simulink model "k1vistmsx"  (Simulink 8.6)
settings: Solver=ode45  StartTime=0.0  StopTime=10.0  RelTol=1e-3
libraries: cdsEpicsOut x52, cdsFilt x39, cdsTP x30, cdsFiltCtrl x26, cdsRms x12, cdsEpicsIn x10, cdsMuxMatrix x6, cdsCDI64 x2, cdsCDO64 x2, cdsIPCx x2, STATE_BIO_MASTER x2, cdsEpicsBinIn x2
(part 1 of 7)
settings Model: Creator=controls  LastModifiedBy=controls
settings OptimizationCC: InitFltsAndDblsToZero=on
settings DebuggingCC: FcnCallInpInsideContextMsg=EnableAllAsWarning  AllowSymbolicDim=on  StrictBusMsg=Warning

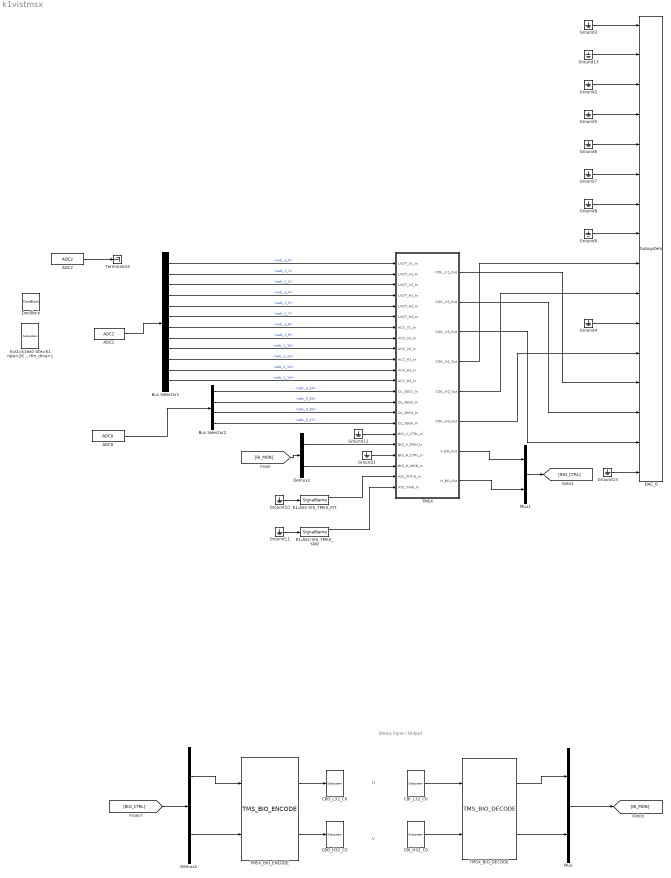
== system k1vistmsx ==
  note: Binary Input / Output
  note: H
  note: V
  ADC0 : cdsAdcx0/ADC0  Tag=cdsAdc  Description=|
      | type-GSC_16AI64SSA
      | card_num=0
      settings: AttributesFormatString=%<Description>\n%<Tag>
  ADC1 : cdsAdcx1/ADC1  Tag=cdsAdc  Description=|
      | type-GSC_16AI64SSA
      | card_num=1
      settings: AttributesFormatString=%<Description>\n%<Tag>
  ADC2 : cdsAdcx2/ADC2  Tag=cdsAdc  Description=|
      | type-GSC_16AI64SSA
      | card_num=2
      settings: AttributesFormatString=%<Description>\n%<Tag>
  Bus Selector1 : BusSelector  Description=ADC Selector  OutputSignals=adc_1_0,adc_1_1,adc_1_2,adc_1_4,adc_1_5,adc_1_7,adc_1_8,adc_1_9,adc_1_10,adc_1_12,adc_1_13,adc_1_14
      settings: AttributesFormatString=%<Description>
  Bus Selector2 : BusSelector  Description=ADC Selector  OutputSignals=adc_0_24,adc_0_25,adc_0_26,adc_0_27
      settings: AttributesFormatString=%<Description>
  CBI_H32_C0 : cdsCDI64/Subsystem  Tag=cdsCDI64  Description=card_num=1
      settings: AttributesFormatString=%<Tag>\n%<Description>
  CBI_L32_C0 : cdsCDI64/Subsystem  Tag=cdsCDI64  Description=card_num=0
      settings: AttributesFormatString=%<Tag>\n%<Description>
  CBO_H32_C0 : cdsCDO64/Subsystem  Tag=cdsCDO64  Description=card_num=1
      settings: AttributesFormatString=%<Tag>\n%<Description>
  CBO_L32_C0 : cdsCDO64/Subsystem  Tag=cdsCDO64  Description=card_num=0
      settings: AttributesFormatString=%<Tag>\n%<Description>
  DAC_0 : dac/Subsystem  Description=|
      | type=GSC_16AO16,
      | card_num=0
      settings: AttributesFormatString=%<Description>
  Demux1 : Demux  Outputs=2
  Demux2 : Demux  Outputs=2
  DocBlock : simulink/Model-Wide Utilities/DocBlock  DocumentType=Text
  Ground{1..13,15} (14 alike) : Ground
  K1:ASC-VIS_TMSX_PIT : cdsIPCx/SignalName  Tag=cdsIPCx_RFM  Description=card=0
      settings: AttributesFormatString=%<Description>\n%<Tag>
  K1:ASC-VIS_TMSX_YAW : cdsIPCx/SignalName  Tag=cdsIPCx_RFM  Description=card=0
      settings: AttributesFormatString=%<Description>\n%<Tag>
  Mux : Mux  Inputs=2
  Mux1 : Mux  Inputs=2
  TMSX : Subsystem  AncestorBlock=VIS_TMS_LIB/TMS_VIS
  TMSX_BIO_DECODE : VIS_TMS_LIB/TMS_BIO_DECODE
  TMSX_BIO_ENCODE : VIS_TMS_LIB/TMS_BIO_ENCODE
  Terminator4 : Terminator
  host=k1ex0 site=K1 rate=2K dcuid=107 specific_cpu=7 adcSlave=1 no_rfm_dma=1 : cdsParameters/Subsystem  Tag=cdsParameters  Description=|
      | Purpose:                                                                                                                                                                                                                                
      |                                                                                                                                                                                                                                         
      | Provide system parameters to the FE code generator to properly configure the generated EPICS names, rep rate of the FE controller, and the Data Acquisition node ID for proper storage of data from this FE controller.                 
      |                                                                                                                                                                                                                                         
      | Useage:                                                                                                                                                                                                                                 
      |                                                                                                                                                                                                                                         
      | The part NAME field is used to identify the FE parameters. It must be of the form:                                                                                                                                                      
      |                                                                                                                                                                                                                                         
      | site=                                                                                                                                                                                                                                   
      | rate=                                                                                                                                                                                                                                   
      | dcuid=                                                                                                                                                                                                                                  
      |                                                                                                                                                                                                                                         
      | Where:                                                                                                                                                                                                                                  
      |                                                                                                                                                                                                                                         
      | site= argument may be H1, H2, L1, M1, G1, either as a single argument or multiple, for example site=H1,H2. These are the only names allowed. These will become the first two characters of all EPICS and signal names (for example G1:).
      |                                                                                                                                                                                                                                         
      | rate= may be 2K, 16K, 32K, or 64K                                                                                                                                                                                                       
      |                                                                                                                                                                                                                                         
      | dcuid= is site specific ie it must be unique at each site.
      settings: AttributesFormatString=%<Tag>
  wires:
  ADC0/1 -> Bus Selector2/1
  Bus Selector1/10 -> TMSX/10(ACC_H1_In)  "<adc_1_12>"
  Bus Selector1/11 -> TMSX/11(ACC_H2_In)  "<adc_1_13>"
  Bus Selector1/12 -> TMSX/12(ACC_H3_In)  "<adc_1_14>"
  TMSX_BIO_ENCODE/1 -> CBO_L32_C0/1
  CBI_L32_C0/1 -> TMSX_BIO_DECODE/1
  TMSX_BIO_DECODE/2 -> Mux/2
  TMSX_BIO_DECODE/1 -> Mux/1
  Mux/1 -> [BI_MON]
  [BIO_CTRL] -> Demux1/1
  TMSX_BIO_ENCODE/2 -> CBO_H32_C0/1
  Demux1/1 -> TMSX_BIO_ENCODE/1
  Demux1/2 -> TMSX_BIO_ENCODE/2
  CBI_H32_C0/1 -> TMSX_BIO_DECODE/2
  [BI_MON] -> Demux2/1
  TMSX/7(V_BO_Out) -> Mux1/1
  TMSX/8(H_BO_Out) -> Mux1/2
  Mux1/1 -> [BIO_CTRL]
  TMSX/1(COIL_V1_Out) -> DAC_0/13
  TMSX/2(COIL_V2_Out) -> DAC_0/14
  TMSX/3(COIL_V3_Out) -> DAC_0/15
  Demux2/1 -> TMSX/18(BIO_V_MON_In)
  Ground1/1 -> TMSX/19(BIO_H_CTRL_In)
  Ground12/1 -> TMSX/17(BIO_V_CTRL_In)
  Demux2/2 -> TMSX/20(BIO_H_MON_In)
  Bus Selector1/1 -> TMSX/1(LVDT_V1_In)  "<adc_1_0>"
  Bus Selector1/2 -> TMSX/2(LVDT_V2_In)  "<adc_1_1>"
  Bus Selector1/3 -> TMSX/3(LVDT_V3_In)  "<adc_1_2>"
  Bus Selector1/4 -> TMSX/4(LVDT_H1_In)  "<adc_1_4>"
  Bus Selector1/5 -> TMSX/5(LVDT_H2_In)  "<adc_1_5>"
  Bus Selector1/6 -> TMSX/6(LVDT_H3_In)  "<adc_1_7>"
  Bus Selector1/7 -> TMSX/7(ACC_V1_In)  "<adc_1_8>"
  Bus Selector1/8 -> TMSX/8(ACC_V2_In)  "<adc_1_9>"
  Bus Selector1/9 -> TMSX/9(ACC_V3_In)  "<adc_1_10>"
  Ground3/1 -> DAC_0/1
  Ground2/1 -> DAC_0/3
  Bus Selector2/1 -> TMSX/13(OL_SEG1_In)  "<adc_0_24>"
  Bus Selector2/2 -> TMSX/14(OL_SEG2_In)  "<adc_0_25>"
  Bus Selector2/3 -> TMSX/15(OL_SEG3_In)  "<adc_0_26>"
  Bus Selector2/4 -> TMSX/16(OL_SEG4_In)  "<adc_0_27>"
  Ground13/1 -> DAC_0/2
  Ground7/1 -> DAC_0/6
  Ground6/1 -> DAC_0/5
  Ground5/1 -> DAC_0/4
  Ground8/1 -> DAC_0/7
  Ground9/1 -> DAC_0/8
  TMSX/4(COIL_H1_Out) -> DAC_0/9
  TMSX/5(COIL_H2_Out) -> DAC_0/10
  Ground4/1 -> DAC_0/11
  TMSX/6(COIL_H3_Out) -> DAC_0/12
  Ground15/1 -> DAC_0/16
  ADC2/1 -> Terminator4/1
  ADC1/1 -> Bus Selector1/1
  Ground10/1 -> K1:ASC-VIS_TMSX_PIT/1
  Ground11/1 -> K1:ASC-VIS_TMSX_YAW/1
  K1:ASC-VIS_TMSX_PIT/1 -> TMSX/21(ASC_PITCH_In)
  K1:ASC-VIS_TMSX_YAW/1 -> TMSX/22(ASC_YAW_In)

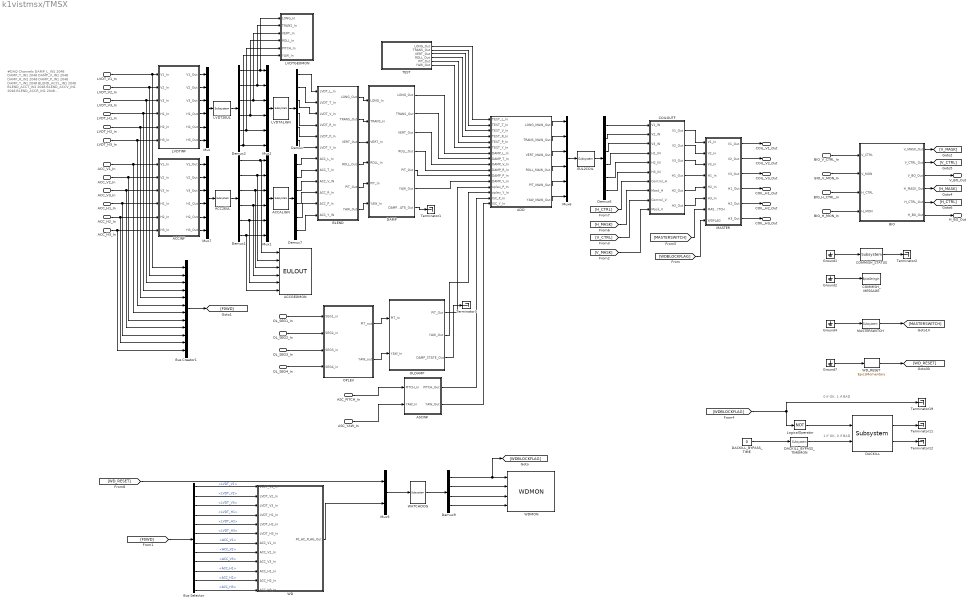
== system k1vistmsx/TMSX ==
  note: #DAQ Channels
      | DAMP_L_IN1 2048
      | DAMP_T_IN1 2048
      | DAMP_V_IN1 2048
      | DAMP_R_IN1 2048
      | DAMP_P_IN1 2048
      | DAMP_Y_IN1 2048
      | BLEND_ACCL_IN1 2048
      | BLEND_ACCT_IN1 2048
      | BLEND_ACCV_IN1 2048
      | BLEND_ACCR_IN1 2048
      | BLEND_ACCP_IN1 2048
      | BLEND_ACCY_IN1 2048
      | BLEND_LVDTL_IN1 2048
      | BLEND_LVDTT_IN1 2048
      | BLEND_LVDTV_IN1 2048
      | BLEND_LVDTR_IN1 2048
      | BLEND_LVDTP_IN1 2048
      | BLEND_LVDTY_IN1 2048
  note: 1 if OK, 0 if BAD
  note: 0 if OK, 1 if BAD
  LVDT_V1_In : Inport
  LVDT_V2_In : Inport  Port=2
  LVDT_V3_In : Inport  Port=3
  LVDT_H1_In : Inport  Port=4
  LVDT_H2_In : Inport  Port=5
  LVDT_H3_In : Inport  Port=6
  ACC_V1_In : Inport  Port=7
  ACC_V2_In : Inport  Port=8
  ACC_V3_In : Inport  Port=9
  ACC_H1_In : Inport  Port=10
  ACC_H2_In : Inport  Port=11
  ACC_H3_In : Inport  Port=12
  OL_SEG1_In : Inport  Port=13
  OL_SEG2_In : Inport  Port=14
  OL_SEG3_In : Inport  Port=15
  OL_SEG4_In : Inport  Port=16
  BIO_V_CTRL_In : Inport  Port=17
  BIO_V_MON_In : Inport  Port=18
  BIO_H_CTRL_In : Inport  Port=19
  BIO_H_MON_In : Inport  Port=20
  ASC_PITCH_In : Inport  Port=21
  ASC_YAW_In : Inport  Port=22
  ACC2EUL : cdsMuxMatrix/Subsystem  Tag=cdsMuxMatrix  Description=|
      | ADL=SUS_INMATRIX.adl 
      | SCRIPT=generate_KisselButton.py 4 5 #CHANNEL# > #TARGET_DIR#/#FULL_PART_NAME#_KB.adl
      settings: AttributesFormatString=%<Tag>
  ACCALIGN : cdsMuxMatrix/Subsystem  Tag=cdsMuxMatrix  Description=Any size matrix. Inputs and outputs must be connected using Mux and Demux parts.
      settings: AttributesFormatString=%<Tag>
  ACCGEOMON : VIS_LIB/EULOUT
  ACCINF : Subsystem
  ADD : Subsystem
  ASCINF : Subsystem
  BIO : Subsystem
  BLEND : Subsystem
  Bus Creator1 : BusCreator  Inputs='LVDT_H1','LVDT_H2','LVDT_H3','LVDT_V1','LVDT_V2','LVDT_V3','ACC_H1','ACC_H2','ACC_H3','ACC_V1','ACC_V2','ACC_V3'
  Bus Selector : BusSelector  OutputSignals=LVDT_V1,LVDT_V2,LVDT_V3,LVDT_H1,LVDT_H2,LVDT_H3,ACC_V1,ACC_V2,ACC_V3,ACC_H1,ACC_H2,ACC_H3
  COILOUTF : Subsystem
  COMMISH_MESSAGE : cdsEpicsStringIn/EpicsStringIn  Tag=cdsEpicsStringIn  Description=cdsEpicsStringIn
      settings: AttributesFormatString=%<Tag>
  COMMISH_STATUS : cdsEpicsBinIn/Subsystem  Tag=cdsEpicsBinIn  Description=|
      | Purpose:                                                                            
      | Create an EPICS binary (0 or 1) input channel to the FE realtime controls.          
      |                                                                                     
      | Operation:                                                                          
      | Outputs value from an EPICS ai record. Value is binary input (bi Epics record type).
      |                                                                                     
      | Usage:                                                                              
      | Name the part with the desired EPICS channel name.
      settings: AttributesFormatString=%<Tag>
  DACKILL : cdsDacKill/Subsystem  Description=cdsDacKill
      settings: AttributesFormatString=%<Description>
  DACKILL_BYPASS_TIME : Constant  Value=0
  DACKILL_BYPASS_TIMEMON : cdsEpicsOut/Subsystem  Tag=cdsEpicsOutput  Description=|
      | Purpose:                                          
      | Output a FE signal to an EPICS channel.           
      |                                                   
      | Operation:                                        
      | Takes input value and passes it to EPICS record.  
      |                                                   
      | Usage:                                            
      | Name the part with the desired EPICS rrecord name.
      settings: AttributesFormatString=%<Tag>
  DAMP : Subsystem
  Demux{,1..2,6..7} (5 alike) : Demux  Outputs=6
  Demux9 : Demux
  EUL2COIL : cdsMuxMatrix/Subsystem  Tag=cdsMuxMatrix  Description=|
      | ADL=SUS_INMATRIX.adl 
      | SCRIPT=generate_KisselButton.py 4 5 #CHANNEL# > #TARGET_DIR#/#FULL_PART_NAME#_KB.adl
      settings: AttributesFormatString=%<Tag>
  Ground{1..2,4,7} (4 alike) : Ground
  LVDT2EUL : cdsMuxMatrix/Subsystem  Tag=cdsMuxMatrix  Description=|
      | ADL=SUS_INMATRIX.adl 
      | SCRIPT=generate_KisselButton.py 4 5 #CHANNEL# > #TARGET_DIR#/#FULL_PART_NAME#_KB.adl
      settings: AttributesFormatString=%<Tag>
  LVDTALIGN : cdsMuxMatrix/Subsystem  Tag=cdsMuxMatrix  Description=Any size matrix. Inputs and outputs must be connected using Mux and Demux parts.
      settings: AttributesFormatString=%<Tag>
  LVDTGEOMON : Subsystem  AncestorBlock=VIS_LIB/EULOUT
  LVDTINF : Subsystem
  LogicalOperator : Logic  Operator=NOT  AllPortsSameDT=off  OutDataTypeStr=boolean
  MASTER : Subsystem
  MASTERSWITCH : cdsEpicsBinIn/Subsystem  Tag=cdsEpicsBinIn  Description=|
      | Purpose:                                                                            
      | Create an EPICS binary (0 or 1) input channel to the FE realtime controls.          
      |                                                                                     
      | Operation:                                                                          
      | Outputs value from an EPICS ai record. Value is binary input (bi Epics record type).
      |                                                                                     
      | Usage:                                                                              
      | Name the part with the desired EPICS channel name.
      settings: AttributesFormatString=%<Tag>
  Mux{,1..2,6..7} (5 alike) : Mux  Inputs=6
  Mux9 : Mux  Inputs=2
  OLDAMP : Subsystem
  OPLEV : Subsystem
  TEST : Subsystem
  Terminator{1..3,11..12,19} (6 alike) : Terminator
  WATCHDOG : cdsFunctionCall/Subsystem  Tag=cdsFunctionCall  Description=inline OSEMWATCHDOG /opt/rtcds/userapps/release/vis/common/src/WATCHDOG.c
      settings: AttributesFormatString=%<Tag>\n%<Description>
  WD : Subsystem
  WDMON : SIXOSEM_F_STAGE_MASTER/SIXOSEM_F_STAGE_MASTER/WDMON
  WD_RESET : cdsEpicsMomentary/EpicsMomentary  Tag=cdsEpicsMomentary
      settings: AttributesFormatString=%<Tag>
  COIL_V1_Out : Outport
  COIL_V2_Out : Outport  Port=2
  COIL_V3_Out : Outport  Port=3
  COIL_H1_Out : Outport  Port=4
  COIL_H2_Out : Outport  Port=5
  COIL_H3_Out : Outport  Port=6
  V_BO_Out : Outport  Port=7
  H_BO_Out : Outport  Port=8
  wires:
  ASCINF/2(YAW_Out) -> ADD/16(ISC_Y_In)
  ASCINF/1(PITCH_Out) -> ADD/15(ISC_P_In)
  ASC_YAW_In/1 -> ASCINF/2(YAW_In)
  ASC_PITCH_In/1 -> ASCINF/1(PITCH_In)
  DAMP/3(VERT_Out) -> ADD/9(DAMP_V_In)
  DAMP/2(TRANS_Out) -> ADD/8(DAMP_T_In)
  DAMP/1(LONG_Out) -> ADD/7(DAMP_L_In)
  TEST/3(VERT_Out) -> ADD/3(TEST_V_In)
  TEST/2(TRANS_Out) -> ADD/2(TEST_T_In)
  TEST/1(LONG_Out) -> ADD/1(TEST_L_In)
  DAMP/7(DAMP_STATE_Out) -> Terminator1/1
  [WDBLOCKFLAG] -> MASTER/8(WDFLAG)
  Bus Creator1/1 -> [F0WD]
  WATCHDOG/1 -> Demux9/1
  Mux9/1 -> WATCHDOG/1
  Demux9/4 -> WDMON/4
  Demux9/3 -> WDMON/3
  Demux9/2 -> WDMON/2
  Demux9/1 -> WDMON/1, [WDBLOCKFLAG]
  [F0WD] -> Bus Selector/1
  WD/1(F0_AC_FLAG_Out) -> Mux9/2
  [WD_RESET] -> Mux9/1
  [MASTERSWITCH] -> MASTER/7(MASTERSWITCH)
  EUL2COIL/1 -> Demux6/1
  Mux6/1 -> EUL2COIL/1
  Demux/3 -> BLEND/3(LVDT_V_In)
  Demux/2 -> BLEND/2(LVDT_T_In)
  Demux/1 -> BLEND/1(LVDT_L_In)
  ACC2EUL/1 -> Demux1/1
  Mux7/1 -> ACC2EUL/1
  LVDT2EUL/1 -> Demux2/1
  Mux/1 -> LVDT2EUL/1
  Demux/4 -> BLEND/4(LVDT_R_In)
  Demux/5 -> BLEND/5(LVDT_P_In)
  Demux/6 -> BLEND/6(LVDT_Y_In)
  Demux7/6 -> BLEND/12(ACC_Y_IN)
  Demux7/5 -> BLEND/11(ACC_P_In)
  Demux7/4 -> BLEND/10(ACC_R_In)
  Demux7/3 -> BLEND/9(ACC_V_IN)
  Demux7/2 -> BLEND/8(ACC_T_In)
  Demux7/1 -> BLEND/7(ACC_L_In)
  BLEND/1(LONG_Out) -> DAMP/1(LONG_In)
  BLEND/2(TRANS_Out) -> DAMP/2(TRANS_In)
  BLEND/3(VERT_Out) -> DAMP/3(VERT_In)
  BLEND/4(ROLL_Out) -> DAMP/4(ROLL_In)
  BLEND/5(PIT_Out) -> DAMP/5(PIT_In)
  BLEND/6(YAW_Out) -> DAMP/6(YAW_In)
  DAMP/4(ROLL_Out) -> ADD/10(DAMP_R_In)
  DAMP/5(PIT_Out) -> ADD/11(DAMP_P_In)
  DAMP/6(YAW_Out) -> ADD/12(DAMP_Y_In)
  TEST/4(ROLL_Out) -> ADD/4(TEST_R_In)
  TEST/5(PIT_Out) -> ADD/5(TEST_P_In)
  TEST/6(YAW_Out) -> ADD/6(TEST_Y_In)
  ADD/1(LONG_MAIN_Out) -> Mux6/1
  ADD/2(TRANS_MAIN_Out) -> Mux6/2
  ADD/3(VERT_MAIN_Out) -> Mux6/3
  ADD/4(ROLL_MAIN_Out) -> Mux6/4
  ADD/5(PIT_MAIN_Out) -> Mux6/5
  ADD/6(YAW_MAIN_Out) -> Mux6/6
  OL_SEG1_In/1 -> OPLEV/1(SEG1_in)
  OL_SEG2_In/1 -> OPLEV/2(SEG2_in)
  OL_SEG3_In/1 -> OPLEV/3(SEG3_in)
  OL_SEG4_In/1 -> OPLEV/4(SEG4_in)
  BIO/1(V_MASK_Out) -> [V_MASK]
  BIO/4(H_MASK_Out) -> [H_MASK]
  BIO/2(V_CTRL_Out) -> [V_CTRL]
  BIO/5(H_CTRL_Out) -> [H_CTRL]
  BIO/3(V_BO_Out) -> V_BO_Out/1
  BIO/6(H_BO_Out) -> H_BO_Out/1
  [H_CTRL] -> COILOUTF/7(Control_H)
  [H_MASK] -> COILOUTF/8(Mask_H)
  [V_CTRL] -> COILOUTF/9(Control_V)
  [V_MASK] -> COILOUTF/10(Mask_V)
  BIO_V_CTRL_In/1 -> BIO/1(V_CTRL)
  BIO_V_MON_In/1 -> BIO/2(V_MON)
  BIO_H_CTRL_In/1 -> BIO/3(H_CTRL)
  BIO_H_MON_In/1 -> BIO/4(H_MON)
  DACKILL/2 -> Terminator12/1
  DACKILL/1 -> Terminator11/1
  DACKILL_BYPASS_TIME/1 -> DACKILL_BYPASS_TIMEMON/1
  DACKILL_BYPASS_TIMEMON/1 -> DACKILL/2
  LogicalOperator/1 -> DACKILL/1
  [WDBLOCKFLAG] -> LogicalOperator/1, Terminator19/1
  Ground1/1 -> COMMISH_STATUS/1
  COMMISH_STATUS/1 -> Terminator2/1
  Ground2/1 -> COMMISH_MESSAGE/1
  MASTERSWITCH/1 -> [MASTERSWITCH]
  Ground4/1 -> MASTERSWITCH/1
  Ground7/1 -> WD_RESET/1
  WD_RESET/1 -> [WD_RESET]
  OPLEV/1(PIT_out) -> OLDAMP/1(PIT_In)
  OPLEV/2(YAW_out) -> OLDAMP/2(YAW_In)
  OLDAMP/1(PIT_Out) -> ADD/13(oplev_P_In)
  OLDAMP/2(YAW_Out) -> ADD/14(oplev_Y_In)
  OLDAMP/3(DAMP_STATE_Out) -> Terminator3/1
  LVDTINF/1(V1_Out) -> Mux/1
  LVDTINF/2(V2_Out) -> Mux/2
  LVDTINF/3(V3_Out) -> Mux/3
  LVDTINF/4(H1_Out) -> Mux/4
  LVDTINF/5(H2_Out) -> Mux/5
  LVDTINF/6(H3_Out) -> Mux/6
  ACCINF/1(V1_Out) -> Mux7/1
  ACCINF/2(V2_Out) -> Mux7/2
  ACCINF/3(V3_Out) -> Mux7/3
  ACCINF/4(H1_Out) -> Mux7/4
  ACCINF/5(H2_Out) -> Mux7/5
  ACCINF/6(H3_Out) -> Mux7/6
  LVDT_V1_In/1 -> LVDTINF/1(V1_In), Bus Creator1/1
  LVDT_V2_In/1 -> LVDTINF/2(V2_In), Bus Creator1/2
  LVDT_V3_In/1 -> LVDTINF/3(V3_In), Bus Creator1/3
  LVDT_H1_In/1 -> LVDTINF/4(H1_In), Bus Creator1/4
  LVDT_H2_In/1 -> LVDTINF/5(H2_In), Bus Creator1/5
  LVDT_H3_In/1 -> LVDTINF/6(H3_In), Bus Creator1/6
  ACC_V1_In/1 -> ACCINF/1(V1_In), Bus Creator1/7
  ACC_V2_In/1 -> ACCINF/2(V2_In), Bus Creator1/8
  ACC_V3_In/1 -> ACCINF/3(V3_In), Bus Creator1/9
  ACC_H1_In/1 -> ACCINF/4(H1_In), Bus Creator1/10
  ACC_H2_In/1 -> ACCINF/5(H2_In), Bus Creator1/11
  ACC_H3_In/1 -> ACCINF/6(H3_In), Bus Creator1/12
  Bus Selector/1 -> WD/1(LVDT_V1_In)  "<LVDT_V1>"
  Bus Selector/2 -> WD/2(LVDT_V2_In)  "<LVDT_V2>"
  Bus Selector/3 -> WD/3(LVDT_V3_In)  "<LVDT_V3>"
  Bus Selector/4 -> WD/4(LVDT_H1_In)  "<LVDT_H1>"
  Bus Selector/5 -> WD/5(LVDT_H2_In)  "<LVDT_H2>"
  Bus Selector/6 -> WD/6(LVDT_H3_In)  "<LVDT_H3>"
  Bus Selector/7 -> WD/7(ACC_V1_In)  "<ACC_V1>"
  Bus Selector/8 -> WD/8(ACC_V2_In)  "<ACC_V2>"
  Bus Selector/9 -> WD/9(ACC_V3_In)  "<ACC_V3>"
  Bus Selector/10 -> WD/10(ACC_H1_In)  "<ACC_H1>"
  Bus Selector/11 -> WD/11(ACC_H2_In)  "<ACC_H2>"
  Bus Selector/12 -> WD/12(ACC_H3_In)  "<ACC_H3>"
  Demux6/1 -> COILOUTF/1(V1_IN)
  Demux6/2 -> COILOUTF/2(V2_IN)
  Demux6/3 -> COILOUTF/3(V3_IN)
  Demux6/4 -> COILOUTF/4(H1_IN)
  Demux6/5 -> COILOUTF/5(H2_IN)
  Demux6/6 -> COILOUTF/6(H3_IN)
  COILOUTF/1(V1_Out) -> MASTER/1(V1_In)
  COILOUTF/2(V2_Out) -> MASTER/2(V2_In)
  COILOUTF/3(V3_Out) -> MASTER/3(V3_In)
  COILOUTF/4(H1_Out) -> MASTER/4(H1_In)
  COILOUTF/5(H2_Out) -> MASTER/5(H2_In)
  COILOUTF/6(H3_Out) -> MASTER/6(H3_In)
  MASTER/1(V1_Out) -> COIL_V1_Out/1
  MASTER/2(V2_Out) -> COIL_V2_Out/1
  MASTER/3(V3_Out) -> COIL_V3_Out/1
  MASTER/4(H1_Out) -> COIL_H1_Out/1
  MASTER/5(H2_Out) -> COIL_H2_Out/1
  MASTER/6(H3_Out) -> COIL_H3_Out/1
  Demux1/1 -> ACCGEOMON/1, Mux1/1
  ACCALIGN/1 -> Demux7/1
  Demux1/2 -> ACCGEOMON/2, Mux1/2
  Demux1/3 -> ACCGEOMON/3, Mux1/3
  Demux1/4 -> ACCGEOMON/4, Mux1/4
  Demux1/5 -> ACCGEOMON/5, Mux1/5
  Demux1/6 -> ACCGEOMON/6, Mux1/6
  Mux1/1 -> ACCALIGN/1
  Demux2/6 -> LVDTGEOMON/6(YAW_In), Mux2/6
  Demux2/4 -> LVDTGEOMON/4(ROLL_In), Mux2/4
  Demux2/3 -> LVDTGEOMON/3(VERT_In), Mux2/3
  Demux2/1 -> LVDTGEOMON/1(LONG_In), Mux2/1
  Mux2/1 -> LVDTALIGN/1
  LVDTALIGN/1 -> Demux/1
  Demux2/2 -> LVDTGEOMON/2(TRANS_In), Mux2/2
  Demux2/5 -> LVDTGEOMON/5(PITCH_In), Mux2/5

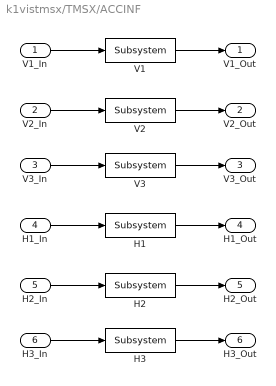
== system k1vistmsx/TMSX/ACCINF ==
  V1_In : Inport
  V2_In : Inport  Port=2
  V3_In : Inport  Port=3
  H1_In : Inport  Port=4
  H2_In : Inport  Port=5
  H3_In : Inport  Port=6
  H1 : cdsFilt/Subsystem  Tag=cdsFilt  Description=|
      | Purpose:                                                                                                                                                                                                                                  
      | Standard CDS IIR filter module.                                                                                                                                                                                                           
      |                                                                                                                                                                                                                                           
      | Operation:                                                                                                                                                                                                                                
      | Consists of 10 second order section IIR filters, plus a ramped gain stage. In FE code, also provides pre-defined test points and excitation channel inputs. The filter coefficients are defined in the LIGO system using the 'foton' tool.
      |                                                                                                                                                                                                                                           
      | Usage:                                                                                                                                                                                                                                    
      | Name the part with the desired filter module name.
      settings: AttributesFormatString=%<Tag>
  H2 : cdsFilt/Subsystem  Tag=cdsFilt  Description=|
      | Purpose:                                                                                                                                                                                                                                  
      | Standard CDS IIR filter module.                                                                                                                                                                                                           
      |                                                                                                                                                                                                                                           
      | Operation:                                                                                                                                                                                                                                
      | Consists of 10 second order section IIR filters, plus a ramped gain stage. In FE code, also provides pre-defined test points and excitation channel inputs. The filter coefficients are defined in the LIGO system using the 'foton' tool.
      |                                                                                                                                                                                                                                           
      | Usage:                                                                                                                                                                                                                                    
      | Name the part with the desired filter module name.
      settings: AttributesFormatString=%<Tag>
  H3 : cdsFilt/Subsystem  Tag=cdsFilt  Description=|
      | Purpose:                                                                                                                                                                                                                                  
      | Standard CDS IIR filter module.                                                                                                                                                                                                           
      |                                                                                                                                                                                                                                           
      | Operation:                                                                                                                                                                                                                                
      | Consists of 10 second order section IIR filters, plus a ramped gain stage. In FE code, also provides pre-defined test points and excitation channel inputs. The filter coefficients are defined in the LIGO system using the 'foton' tool.
      |                                                                                                                                                                                                                                           
      | Usage:                                                                                                                                                                                                                                    
      | Name the part with the desired filter module name.
      settings: AttributesFormatString=%<Tag>
  V1 : cdsFilt/Subsystem  Tag=cdsFilt  Description=|
      | Purpose:                                                                                                                                                                                                                                  
      | Standard CDS IIR filter module.                                                                                                                                                                                                           
      |                                                                                                                                                                                                                                           
      | Operation:                                                                                                                                                                                                                                
      | Consists of 10 second order section IIR filters, plus a ramped gain stage. In FE code, also provides pre-defined test points and excitation channel inputs. The filter coefficients are defined in the LIGO system using the 'foton' tool.
      |                                                                                                                                                                                                                                           
      | Usage:                                                                                                                                                                                                                                    
      | Name the part with the desired filter module name.
      settings: AttributesFormatString=%<Tag>
  V2 : cdsFilt/Subsystem  Tag=cdsFilt  Description=|
      | Purpose:                                                                                                                                                                                                                                  
      | Standard CDS IIR filter module.                                                                                                                                                                                                           
      |                                                                                                                                                                                                                                           
      | Operation:                                                                                                                                                                                                                                
      | Consists of 10 second order section IIR filters, plus a ramped gain stage. In FE code, also provides pre-defined test points and excitation channel inputs. The filter coefficients are defined in the LIGO system using the 'foton' tool.
      |                                                                                                                                                                                                                                           
      | Usage:                                                                                                                                                                                                                                    
      | Name the part with the desired filter module name.
      settings: AttributesFormatString=%<Tag>
  V3 : cdsFilt/Subsystem  Tag=cdsFilt  Description=|
      | Purpose:                                                                                                                                                                                                                                  
      | Standard CDS IIR filter module.                                                                                                                                                                                                           
      |                                                                                                                                                                                                                                           
      | Operation:                                                                                                                                                                                                                                
      | Consists of 10 second order section IIR filters, plus a ramped gain stage. In FE code, also provides pre-defined test points and excitation channel inputs. The filter coefficients are defined in the LIGO system using the 'foton' tool.
      |                                                                                                                                                                                                                                           
      | Usage:                                                                                                                                                                                                                                    
      | Name the part with the desired filter module name.
      settings: AttributesFormatString=%<Tag>
  V1_Out : Outport
  V2_Out : Outport  Port=2
  V3_Out : Outport  Port=3
  H1_Out : Outport  Port=4
  H2_Out : Outport  Port=5
  H3_Out : Outport  Port=6
  wires:
  H3/1 -> H3_Out/1
  H3_In/1 -> H3/1
  H2/1 -> H2_Out/1
  H2_In/1 -> H2/1
  H1/1 -> H1_Out/1
  H1_In/1 -> H1/1
  V3/1 -> V3_Out/1
  V3_In/1 -> V3/1
  V2/1 -> V2_Out/1
  V2_In/1 -> V2/1
  V1/1 -> V1_Out/1
  V1_In/1 -> V1/1

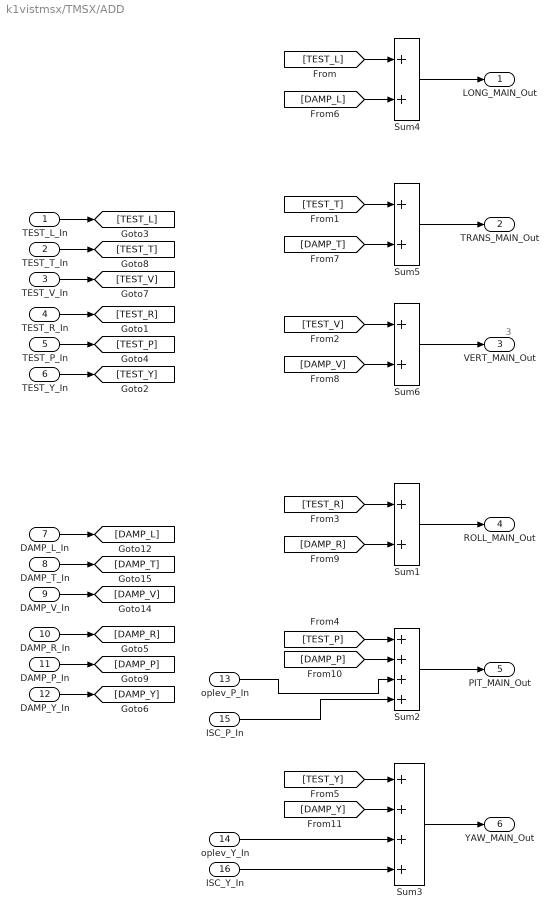
== system k1vistmsx/TMSX/ADD ==
  note: 3
  TEST_L_In : Inport
  TEST_T_In : Inport  Port=2
  TEST_V_In : Inport  Port=3
  TEST_R_In : Inport  Port=4
  TEST_P_In : Inport  Port=5
  TEST_Y_In : Inport  Port=6
  DAMP_L_In : Inport  Port=7
  DAMP_T_In : Inport  Port=8
  DAMP_V_In : Inport  Port=9
  DAMP_R_In : Inport  Port=10
  DAMP_P_In : Inport  Port=11
  DAMP_Y_In : Inport  Port=12
  oplev_P_In : Inport  Port=13
  oplev_Y_In : Inport  Port=14
  ISC_P_In : Inport  Port=15
  ISC_Y_In : Inport  Port=16
  Sum{1,4..6} (4 alike) : Sum
  Sum2 : Sum  Inputs=++++
  Sum3 : Sum  Inputs=++++
  LONG_MAIN_Out : Outport
  TRANS_MAIN_Out : Outport  Port=2
  VERT_MAIN_Out : Outport  Port=3
  ROLL_MAIN_Out : Outport  Port=4
  PIT_MAIN_Out : Outport  Port=5
  YAW_MAIN_Out : Outport  Port=6
  wires:
  ISC_Y_In/1 -> Sum3/4
  ISC_P_In/1 -> Sum2/4
  oplev_Y_In/1 -> Sum3/3
  Sum3/1 -> YAW_MAIN_Out/1
  Sum2/1 -> PIT_MAIN_Out/1
  DAMP_V_In/1 -> [DAMP_V]
  DAMP_T_In/1 -> [DAMP_T]
  DAMP_L_In/1 -> [DAMP_L]
  TEST_V_In/1 -> [TEST_V]
  TEST_T_In/1 -> [TEST_T]
  TEST_L_In/1 -> [TEST_L]
  Sum1/1 -> ROLL_MAIN_Out/1
  TEST_Y_In/1 -> [TEST_Y]
  TEST_P_In/1 -> [TEST_P]
  TEST_R_In/1 -> [TEST_R]
  Sum5/1 -> TRANS_MAIN_Out/1
  Sum4/1 -> LONG_MAIN_Out/1
  Sum6/1 -> VERT_MAIN_Out/1
  DAMP_Y_In/1 -> [DAMP_Y]
  DAMP_P_In/1 -> [DAMP_P]
  DAMP_R_In/1 -> [DAMP_R]
  [TEST_L] -> Sum4/1
  [TEST_T] -> Sum5/1
  [TEST_V] -> Sum6/1
  [TEST_R] -> Sum1/1
  [TEST_P] -> Sum2/1
  [TEST_Y] -> Sum3/1
  [DAMP_L] -> Sum4/2
  [DAMP_T] -> Sum5/2
  [DAMP_V] -> Sum6/2
  [DAMP_R] -> Sum1/2
  [DAMP_P] -> Sum2/2
  [DAMP_Y] -> Sum3/2
  oplev_P_In/1 -> Sum2/3

== system k1vistmsx/TMSX/ASCINF ==
  PITCH_In : Inport
  YAW_In : Inport  Port=2
  P : cdsFilt/Subsystem  Tag=cdsFilt  Description=|
      | Purpose:                                                                                                                                                                                                                                  
      | Standard CDS IIR filter module.                                                                                                                                                                                                           
      |                                                                                                                                                                                                                                           
      | Operation:                                                                                                                                                                                                                                
      | Consists of 10 second order section IIR filters, plus a ramped gain stage. In FE code, also provides pre-defined test points and excitation channel inputs. The filter coefficients are defined in the LIGO system using the 'foton' tool.
      |                                                                                                                                                                                                                                           
      | Usage:                                                                                                                                                                                                                                    
      | Name the part with the desired filter module name.
      settings: AttributesFormatString=%<Tag>
  Y : cdsFilt/Subsystem  Tag=cdsFilt  Description=|
      | Purpose:                                                                                                                                                                                                                                  
      | Standard CDS IIR filter module.                                                                                                                                                                                                           
      |                                                                                                                                                                                                                                           
      | Operation:                                                                                                                                                                                                                                
      | Consists of 10 second order section IIR filters, plus a ramped gain stage. In FE code, also provides pre-defined test points and excitation channel inputs. The filter coefficients are defined in the LIGO system using the 'foton' tool.
      |                                                                                                                                                                                                                                           
      | Usage:                                                                                                                                                                                                                                    
      | Name the part with the desired filter module name.
      settings: AttributesFormatString=%<Tag>
  PITCH_Out : Outport
  YAW_Out : Outport  Port=2
  wires:
  Y/1 -> YAW_Out/1
  P/1 -> PITCH_Out/1
  YAW_In/1 -> Y/1
  PITCH_In/1 -> P/1

== system k1vistmsx/TMSX/BIO ==
  V_CTRL : Inport
  V_MON : Inport  Port=2
  H_CTRL : Inport  Port=3
  H_MON : Inport  Port=4
  H : STATE_BIO_MASTER/UIM_BIO_MASTER
  V : STATE_BIO_MASTER/UIM_BIO_MASTER
  V_MASK_Out : Outport
  V_CTRL_Out : Outport  Port=2
  V_BO_Out : Outport  Port=3
  H_MASK_Out : Outport  Port=4
  H_CTRL_Out : Outport  Port=5
  H_BO_Out : Outport  Port=6
  wires:
  H/2 -> H_CTRL_Out/1
  H/1 -> H_MASK_Out/1
  V/1 -> V_MASK_Out/1
  H_MON/1 -> H/2
  H_CTRL/1 -> H/1
  H/3 -> H_BO_Out/1
  V_CTRL/1 -> V/1
  V/2 -> V_CTRL_Out/1
  V_MON/1 -> V/2
  V/3 -> V_BO_Out/1
